simulink model "battery_soc"  (R2023a)
settings: Solver=VariableStepAuto  StartTime=0.0  StopTime=Tf*n  RelTol=1e-3
values from neighbouring files (symbols this model uses):
  n = 200    [main.m]
  Te = 1    [main.m]
  Vo = 4.2    [main.m]
libraries: fl_lib x7, nesl_utility x7, simulink x1
settings Model: Creator=dmm  LastModifiedBy=dmm
settings OptimizationCC: ReuseModelBlockBuffer=off

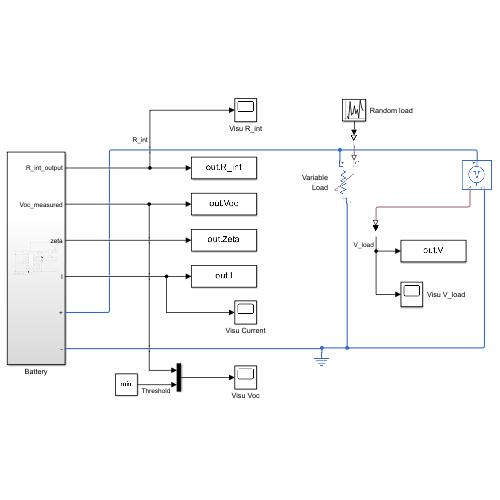
[thumbnail: Simulink's stored preview of the top-level diagram]
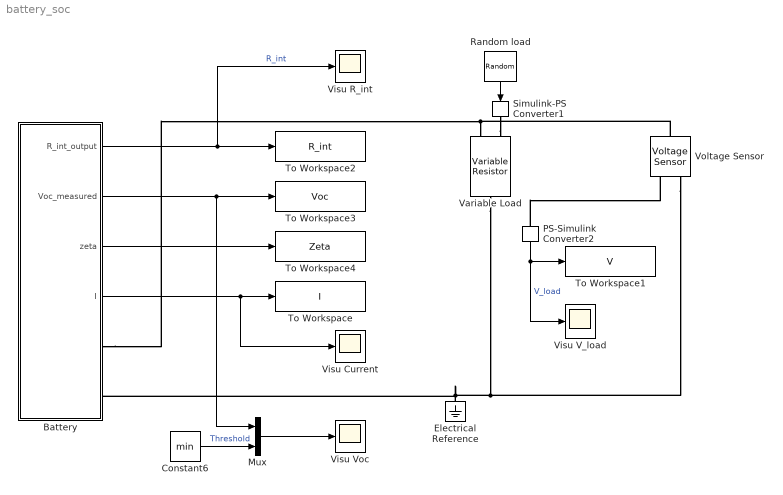
== system battery_soc ==
  Battery : Subsystem
  Constant6 : Constant  Value=min
  Electrical Reference : fl_lib/Electrical/Electrical Elements/Electrical Reference
  Mux : Mux  Inputs=2
  PS-Simulink Converter2 : nesl_utility/PS-Simulink Converter  PhysicalDomain=network_engine_domain  SubClassName=ps_output  LeftPortType=input  RightPortType=output  PseudoPeriodic=off  Frequencies=[]  VectorFormat=inherit  Unit=inherit  AffineConversion=off
  Random load : UniformRandomNumber  Minimum=3  Maximum=5  Seed=randi(100)  SampleTime=0.1
  Simulink-PS Converter1 : nesl_utility/Simulink-PS Converter  PhysicalDomain=network_engine_domain  SubClassName=ps_input  LeftPortType=input  RightPortType=output  PseudoPeriodic=off  Frequencies=[]  NoiseDistribution=none  NoiseParameters=[]  Unit=1  AffineConversion=off  FilteringAndDerivatives=provide  SimscapeFilterOrder=1  InputFilterTimeConstant=0.001  UdotUserProvided=0
  To Workspace : ToWorkspace  VariableName=I  SaveFormat=Structure With Time  SampleTime=-1
  To Workspace1 : ToWorkspace  VariableName=V  SaveFormat=Structure With Time  SampleTime=-1
  To Workspace2 : ToWorkspace  VariableName=R_int  SaveFormat=Structure With Time  SampleTime=-1
  To Workspace3 : ToWorkspace  VariableName=Voc  SaveFormat=Structure With Time  SampleTime=-1
  To Workspace4 : ToWorkspace  VariableName=Zeta  SaveFormat=Structure With Time  SampleTime=-1
  Variable Load : fl_lib/Electrical/Electrical Elements/Variable Resistor  Rmin=0 Ohm  i_specify=off  i_priority=None  i=0 A  i_nominal_specify=off  i_nominal_unit=A  i_nominal_value=1  v_specify=off  v_priority=None  v=0 V  v_nominal_specify=off  v_nominal_unit=V  v_nominal_value=1
  Visu Current : Scope
  Visu R_int : Scope
  Visu V_load : Scope
  Visu Voc : Scope
  Voltage Sensor : fl_lib/Electrical/Electrical Sensors/Voltage Sensor
  wires:
  Random load/1 -> Simulink-PS Converter1/1
  PS-Simulink Converter2/1 -> Visu V_load/1, To Workspace1/1  "V_load"
  Constant6/1 -> Mux/2  "Threshold"
  Mux/1 -> Visu Voc/1
  Battery/2(Voc_measured) -> To Workspace3/1, Mux/1
  Battery/3(zeta) -> To Workspace4/1
  Battery/4(I) -> Visu Current/1, To Workspace/1
  Battery/1(R_int_output) -> Visu R_int/1, To Workspace2/1  "R_int"
  connections:
  Simulink-PS Converter1/RConn1 -- Variable Load/LConn1
  Voltage Sensor/LConn1 -- Battery/RConn1 -- Variable Load/LConn2
  PS-Simulink Converter2/LConn1 -- Voltage Sensor/RConn1
  Variable Load/RConn1 -- Voltage Sensor/RConn2 -- Electrical Reference/LConn1 -- Battery/RConn2

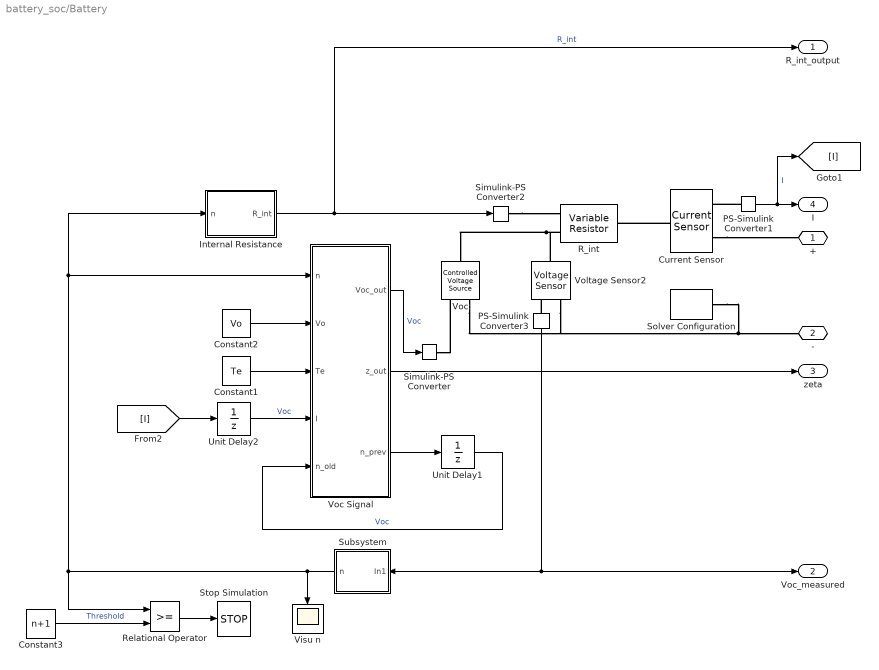
== system battery_soc/Battery ==
  Constant1 : Constant  Value=Te
  Constant2 : Constant  Value=Vo
  Constant3 : Constant  Value=n+1
  Current Sensor : fl_lib/Electrical/Electrical Sensors/Current Sensor
  Internal Resistance : MATLAB Function  TreatAsAtomicUnit=on
  PS-Simulink Converter1 : nesl_utility/PS-Simulink Converter  PhysicalDomain=network_engine_domain  SubClassName=ps_output  LeftPortType=input  RightPortType=output  PseudoPeriodic=off  Frequencies=[]  VectorFormat=inherit  Unit=inherit  AffineConversion=off
  PS-Simulink Converter3 : nesl_utility/PS-Simulink Converter  PhysicalDomain=network_engine_domain  SubClassName=ps_output  LeftPortType=input  RightPortType=output  PseudoPeriodic=off  Frequencies=[]  VectorFormat=inherit  Unit=inherit  AffineConversion=off
  R_int : fl_lib/Electrical/Electrical Elements/Variable Resistor  Rmin=0 Ohm  i_specify=off  i_priority=None  i=0 A  i_nominal_specify=off  i_nominal_unit=A  i_nominal_value=1  v_specify=off  v_priority=None  v=0 V  v_nominal_specify=off  v_nominal_unit=V  v_nominal_value=1
  Relational Operator : RelationalOperator  OutDataTypeStr=boolean  RndMeth=Simplest  InputSameDT=off
  Simulink-PS Converter : nesl_utility/Simulink-PS Converter  PhysicalDomain=network_engine_domain  SubClassName=ps_input  LeftPortType=input  RightPortType=output  PseudoPeriodic=off  Frequencies=[]  NoiseDistribution=none  NoiseParameters=[]  Unit=1  AffineConversion=off  FilteringAndDerivatives=provide  SimscapeFilterOrder=1  InputFilterTimeConstant=0.001  UdotUserProvided=0
  Simulink-PS Converter2 : nesl_utility/Simulink-PS Converter  PhysicalDomain=network_engine_domain  SubClassName=ps_input  LeftPortType=input  RightPortType=output  PseudoPeriodic=off  Frequencies=[]  NoiseDistribution=none  NoiseParameters=[]  Unit=1  AffineConversion=off  FilteringAndDerivatives=provide  SimscapeFilterOrder=1  InputFilterTimeConstant=0.001  UdotUserProvided=0
  Solver Configuration : nesl_utility/Solver Configuration  PhysicalDomain=network_engine_domain  SubClassName=solver  LeftPortType=input  RightPortType=generic  Tones=[]  Harmonics=[]  SimulateNoise=off  Profile=off  UseLocalSampling=off  EnableSwitchedLinearOptims=on  FrequencyDomain=off  UseCCode=off  RelTol=0.001  AbsTol=0.001  MinStep=1e-09  ToWorkspace=off  RevertToSquareIcSolve=off  NumHomotopyIterations=100  PhasorMode=off  PhasorModeNumHarmonics=1  ConsistencySolver=NEWTON_XTOL_AFTER_FTOL  IndexReductionMethod=DerivativeReplacement  DoDC=off  ResidualTolerance=1e-09  ConsistencyTolSource=GLOBAL  ConsistencyAbsTol=0.001  ConsistencyRelTol=0.001  ConsistencyTolFactor=0.001  UseLocalSolver=off  LocalSolverChoice=NE_BACKWARD_EULER_ADVANCER  ResolveIndetEquations=on  FunctionEvalNumThread=1  LocalSolverSampleTime=0.001  DoFixedCost=off  MaxNonlinIter=3  MaxModeIter=2  ComputeImpulses=off  ImpulseIterations=2  LinearAlgebra=auto  LinearAlgebraNumThread=0  EquationFormulation=NE_TIME_EF  DelaysMemoryBudget=1024  AutomaticFiltering=on  FilteringTimeConstant=0.001  PartitionStorageMethod=AS_NEEDED  PartitionMemoryBudget=1024  PartitionMethod=ROBUST
  Stop Simulation : Stop
  Subsystem : Subsystem
  Unit Delay1 : UnitDelay  SampleTime=-1  HasFrameUpgradeWarning=on
  Unit Delay2 : UnitDelay  SampleTime=-1  HasFrameUpgradeWarning=on
  Visu n : Scope
  Voc : fl_lib/Electrical/Electrical Sources/Controlled Voltage Source
  Voc Signal : MATLAB Function  TreatAsAtomicUnit=on
  Voltage Sensor2 : fl_lib/Electrical/Electrical Sensors/Voltage Sensor
  + : PMIOPort  Side=Right
  - : PMIOPort  Port=2  Side=Right
  R_int_output : Outport
  Voc_measured : Outport  Port=2
  zeta : Outport  Port=3
  I : Outport  Port=4
  wires:
  Unit Delay2/1 -> Voc Signal/4(I)  "Voc"
  Voc Signal/3(n_prev) -> Unit Delay1/1
  [I] -> Unit Delay2/1
  Constant3/1 -> Relational Operator/2  "Threshold"
  Unit Delay1/1 -> Voc Signal/5(n_old)  "Voc"
  Voc Signal/1(Voc_out) -> Simulink-PS Converter/1  "Voc"
  Voc Signal/2(z_out) -> zeta/1
  Subsystem/1(n) -> Visu n/1, Relational Operator/1, Internal Resistance/1(n), Voc Signal/1(n)
  Relational Operator/1 -> Stop Simulation/1
  Constant2/1 -> Voc Signal/2(Vo)
  Internal Resistance/1(R_int) -> R_int_output/1, Simulink-PS Converter2/1  "R_int"
  PS-Simulink Converter3/1 -> Voc_measured/1, Subsystem/1(In1)
  Constant1/1 -> Voc Signal/3(Te)
  PS-Simulink Converter1/1 -> [I], I/1  "I"
  connections:
  R_int/LConn2 -- Voltage Sensor2/LConn1 -- Voc/LConn1
  Current Sensor/RConn2 -- +/RConn1
  PS-Simulink Converter3/LConn1 -- Voltage Sensor2/RConn1
  Current Sensor/LConn1 -- R_int/RConn1
  Simulink-PS Converter2/RConn1 -- R_int/LConn1
  Simulink-PS Converter/RConn1 -- Voc/RConn1
  PS-Simulink Converter1/LConn1 -- Current Sensor/RConn1
  Solver Configuration/RConn1 -- Voc/RConn2 -- Voltage Sensor2/RConn2 -- -/RConn1

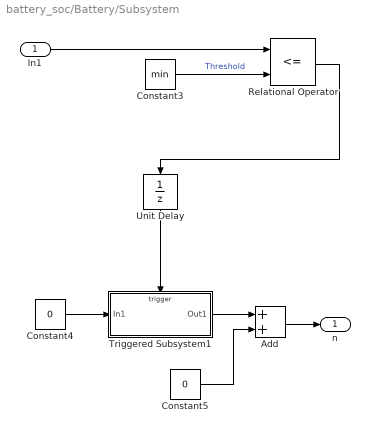
== system battery_soc/Battery/Subsystem ==
  In1 : Inport
  Add : Sum
  Constant3 : Constant  Value=min
  Constant4 : Constant  Value=0
  Constant5 : Constant  Value=0
  Relational Operator : RelationalOperator  Operator=<=  OutDataTypeStr=boolean  RndMeth=Simplest  InputSameDT=off
  Triggered Subsystem1 : Subsystem  TreatAsAtomicUnit=on
  Unit Delay : UnitDelay  SampleTime=-1  HasFrameUpgradeWarning=on
  n : Outport
  wires:
  Relational Operator/1 -> Unit Delay/1
  Unit Delay/1 -> Triggered Subsystem1/Trigger
  Constant3/1 -> Relational Operator/2  "Threshold"
  Triggered Subsystem1/1(Out1) -> Add/1
  Constant5/1 -> Add/2
  In1/1 -> Relational Operator/1
  Constant4/1 -> Triggered Subsystem1/1(In1)
  Add/1 -> n/1

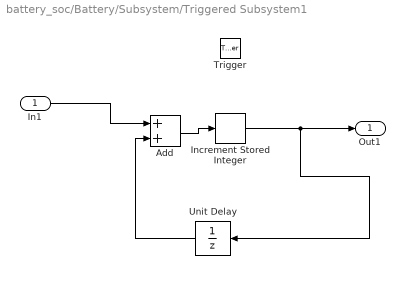
== system battery_soc/Battery/Subsystem/Triggered Subsystem1 ==
  In1 : Inport  OutDataTypeStr=double  LockScale=on
  Trigger : TriggerPort  VariantControl=(inherit)
  Add : Sum
  Increment Stored Integer : simulink/Additional Math & Discrete/Additional Math: Increment - Decrement/Increment Stored Integer
  Unit Delay : UnitDelay  SampleTime=-1  HasFrameUpgradeWarning=on
  Out1 : Outport
  wires:
  Increment Stored Integer/1 -> Out1/1, Unit Delay/1
  In1/1 -> Add/1
  Add/1 -> Increment Stored Integer/1
  Unit Delay/1 -> Add/2

== matlab function battery_soc/Battery/Voc Signal ==
  data: n input; Vo input; Voc_out output; z_out output; Te input; I input; n_old input; n_prev output
function [Voc_out, z_out, n_prev] = fcn(n, Vo, Te, I, n_old)
    persistent z
    persistent Voc

    if isempty(n_old)
        n_prev = 0;
    end
    
    if n == n_old + 1
        z = 100;
        Voc = Vo;
    end
    

    if isempty(z)
        z = 100;
    end

    if isempty(Voc)
        Voc = Vo;
    end

    
    K1 = 0.07;
    K2 = 0.7;


    Cn = 2; %[Ah]
    Cr = Cn - 0.1*n; %Loss of the SoC based in the n cycles

    z = z - Te*I*(100 / (3600*Cr));
    z_out = z;

    y = Vo -K1*log(100 - z ) - K2 / z;
    y = min(y, 4.2);
    
    alpha = exp(-Te/90);
    Voc = alpha*Voc + (1-alpha)*y;
    Voc_out = Voc;
    n_prev = n;

end

== matlab function battery_soc/Battery/Internal Resistance ==
  data: n input; R_int output
function R_int = fcn(n)
    R_int = 0.06 + 8.4375E-5*n;
end
